simulink model "mpc_tmpdemo2"  (R2015a)
settings: Solver=ode45  SolverMode=SingleTasking  StartTime=0.0  StopTime=20.0  RelTol=1e-3
PreLoadFcn:
  | load mpc_tmpdemodata;
  | mpctmpinit
undefined symbols (not defined in the file or in its folder): Fb0, Fbh0, iA, ke, ke2, kf, kf2, lastu, lastx, m2, M2, MVscale, nv, nym, p, Rscale, st, ts, uoff, xoff
libraries: mpcsigdimcheck_private x14, cstblocks x9, simulink x4
settings Model: FPTRunName=Active  CovSFcnEnable=off  Creator=The MathWorks Inc.  LastModifiedBy=Yi
settings OptimizationCC: BlockReduction=off  BooleanDataType=off
settings DebuggingCC: SaveWithParameterizedLinksMsg=none  UnderspecifiedInitializationDetection=Classic  MergeDetectMultiDrivingBlocksExec=none  SignalResolutionControl=TryResolveAllWithWarning
settings HardwareCC: TargetUnknown=on

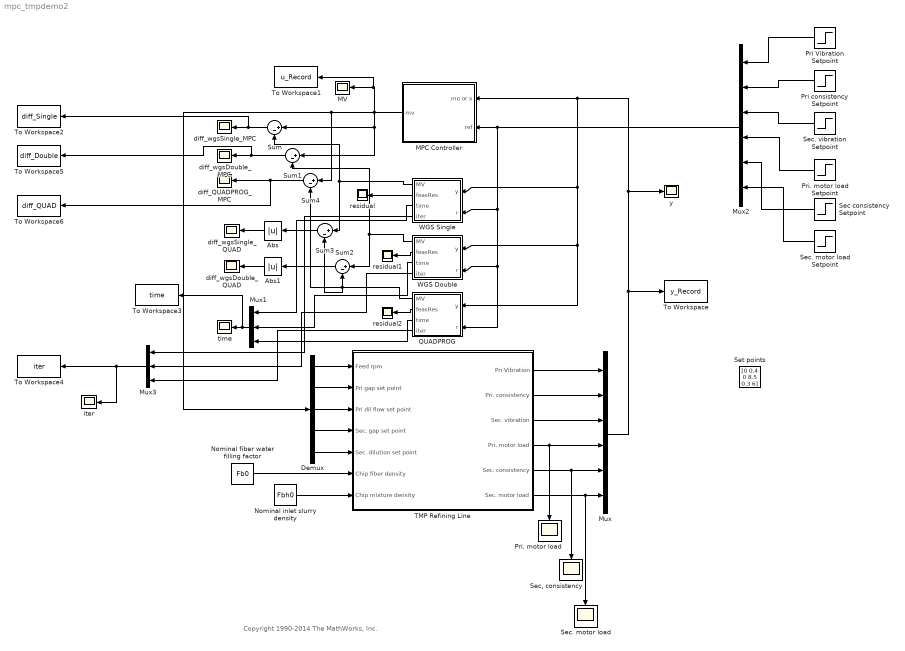
== system mpc_tmpdemo2 ==
  note: Copyright 1990-2014 The MathWorks, Inc.
  " residual" : Scope
      settings: TimeRange=7  YMin=-0.05  YMax=0.15  SaveName=ScopeData4  DataFormat=Structure
  " residual1" : Scope
      settings: TimeRange=7  YMin=-0.05  YMax=0.15  SaveName=ScopeData9  DataFormat=Structure
  " residual2" : Scope
      settings: TimeRange=7  YMin=-0.05  YMax=0.15  SaveName=ScopeData10  DataFormat=Structure
  Abs : Abs
  Abs1 : Abs
  Demux : Demux  Outputs=5
  MPC Controller : Subsystem  AncestorBlock=mpclib/MPC Controller  InitFcn=impcblock_InitFcn  StartFcn=impcblock_StartFcn  mask(MPC){mpcobj=mpcobj, x0=[], is_multiple=0, enable_value=0, n_mv=5, n_mo=6, n_md=0, n_ts=0.5, is_designfromscratch=0, return_u0=off, ref_from_ws=off, ref_signal_name=[], ref_preview=on, md_from_ws=off, md_signal_name=[], md_preview=on, from_project=off, project_file=MPCtask.mat, project_name=, task_name=, md_inport=off, mv_inport=off, cost_outport=off, return_sequence=off, return_qpstatus=off, return_state=off, state_inport=off, lims_inport=off, ywt_inport=off, uwt_inport=off, duwt_inport=off, rhoeps_inport=off, uref_inport=off, BlockDataType=double, SampleTimeInherited=off, switch_inport=off}
      mask prompts: mpcobj "MPC:general:BlgIMPC"; x0 "MPC:general:BlgState"; is_multiple "Flag indicating the block is part of multiple blocks"; enable_value "Value enabling optimization"; n_mv "Number of MVs"; n_mo "Number of MOs"; n_md "Number of MDs"; n_ts "Sample Time"; is_designfromscratch "Design from scratch flag"; return_u0 "Export u0"; ref_from_ws "Obsolete"; ref_signal_name "Obsolete"; ref_preview "Obsolete"; md_from_ws "Obsolete"; md_signal_name "Obsolete"; md_preview "Obsolete"; from_project "Obsolete"; project_file "Obsolete"; project_name "Obsolete"; task_name "Obsolete"; md_inport "MPC:general:BlgMD"; mv_inport "MPC:general:BlgEXTMV"; cost_outport "MPC:general:BlgCOST"; return_sequence "MPC:general:BlgMVSEQ"; return_qpstatus "MPC:general:BlgQPSTATUS"; return_state "MPC:general:BlgESTSTATE"; state_inport "MPC:general:BlgXKK"; lims_inport "MPC:general:BlgLIMITS"; ywt_inport "MPC:general:BlgYWT"; uwt_inport "MPC:general:BlgUWT"; duwt_inport "MPC:general:BlgDUWT"; rhoeps_inport "MPC:general:BlgECRWT"; uref_inport "MPC:general:BlgMVTARGET"; BlockDataType "MPC:general:BlgDATATYPE"; SampleTimeInherited "MPC:general:BlgTS"; switch_inport "MPC:general:BlgSWITCH"
      mask help: MPC:utility:MaskDescMPC1
      mask init:
      | [blk,ts,A,Cm,Bu,Bv,Dvm,isQP,strmoorx,nmoorx,nu,nv,ny,nx,nym...
      |     degrees,L,M,H,Hinv,Linv,iA,Ac,Kx,Ku1,Kut,Kr,Kv,...
      |     Mlim,Mx,Mu1,Mv,z_degrees,utarget,...
      |     lastx,lastu,p,xoff,uoff,yoff,voff,myoff,no_md,no_ref,...
      |     maxiter,nxQP,openloopflag,no_ym,...
      |     lims_inport,no_umin,no_umax,no_ymin,no_ymax,...
      |     switch_inport,no_switch,enable_value,...
      |     return_cost,return_sequence,CustomEstimation,...
      |     no_ywt, no_uwt, no_duwt, no_rhoeps, no_uref, no_mv, ...
      |     Wy,Wdu,Jm,SuJm,Su1,Sx,Hv,Wu,I1,...
      |     isAdaptive, C, Dv, Mrows, nCC, Ecc, Fcc, Scc, Gcc, ...
      |     Uscale, Yscale, nxp, nxindist, mvindex, mdindex, unindex,  ...
      |     myindex,Rscale,MVscale,MDscale] = impcblock_MaskInitFcnParameter();
      | impcblock_MaskInitFcnResize(gcb,nv,nu,ny);
      settings: DeleteFcn=impcblock_DeleteFcn
      mask Help: eval('mpcCSHelp(''MPCmask'',''HelpBrowser'')');
      mask Callback state_inport: mpc_blockdialogcallback(gcb);
      mask DialogControl design_button Prompt: MPC:general:BlgDesignButton
      mask DialogControl design_button Callback: mpc_designcallback(gcbh)
      mask DialogControl review_button Prompt: MPC:general:BlgReviewButton
      mask DialogControl review_button Callback: mpc_reviewcallback(gcbh)
      mask Display:
      | fprintf('MPC');
      | port_label('output', 1, 'mv')
      | port_label('input', 1, 'mo')
      | port_label('input', 2, 'ref')
  MV : Scope
      settings: SaveName=ScopeData6
  Mux : Mux  Inputs=6
  Mux1 : Mux  Inputs=3
  Mux2 : Mux  Inputs=6
  Mux3 : Mux  Inputs=3
  Nominal fiber water filling factor : Constant  Value=Fb0
  Nominal inlet slurry density : Constant  Value=Fbh0
  Pri Vibration Setpoint : Step  Time=0  After=0  SampleTime=0
  Pri consistency Setpoint : Step  Before=0.5  After=0.5  SampleTime=0
  Pri. motor load : Scope
      settings: YMin=0.3825  YMax=0.415
  Pri. motor load Setpoint : Step  Time=0  Before=8.5  After=8.5  SampleTime=0
  QUADPROG : Subsystem
  Sec consistency Setpoint : Step  Time=0  Before=0.4  After=0.4  SampleTime=0
  "Sec, consistency" : Scope
      settings: YMin=0.3825  YMax=0.415
  Sec. motor load : Scope
      settings: YMin=0.3825  YMax=0.415  SaveName=ScopeData2
  Sec. motor load Setpoint : Step  Time=0  Before=7  After=7  SampleTime=0
  Sec. vibration Setpoint : Step  Time=0  After=0  SampleTime=0
  Set points : Constant  Value=[0 0.4 0 8.5 0.3 6]
  Sum{,1..4} (5 alike) : Sum  Inputs=|+-
  TMP Refining Line : Subsystem
  To Workspace : ToWorkspace  VariableName=y_Record  SampleTime=-1
  To Workspace1 : ToWorkspace  VariableName=u_Record  SampleTime=-1
  To Workspace2 : ToWorkspace  VariableName=diff_Single  SampleTime=-1
  To Workspace3 : ToWorkspace  VariableName=time  SampleTime=-1
  To Workspace4 : ToWorkspace  VariableName=iter  SampleTime=-1
  To Workspace5 : ToWorkspace  VariableName=diff_Double  SampleTime=-1
  To Workspace6 : ToWorkspace  VariableName=diff_QUAD  SampleTime=-1
  WGS Double : Subsystem
  WGS Single : Subsystem
  diff_QUADPROG_MPC : Scope
      settings: SaveName=ScopeData14
  diff_wgsDouble_MPC : Scope
      settings: SaveName=ScopeData5
  diff_wgsDouble_QUAD : Scope
      settings: SaveName=ScopeData11
  diff_wgsSingle_MPC : Scope
      settings: SaveName=ScopeData3
  diff_wgsSingle_QUAD : Scope
      settings: SaveName=ScopeData12
  iter : Scope
      settings: SaveName=ScopeData16
  time : Scope
      settings: SaveName=ScopeData13
  y : Scope
      settings: SaveName=ScopeData15
  wires:
  Demux/1 -> TMP Refining Line/1(Feed rpm)
  Demux/3 -> TMP Refining Line/3(Pri dil flow set point)
  Demux/4 -> TMP Refining Line/4(Sec. gap set point)
  Demux/5 -> TMP Refining Line/5(Sec. dilution set point)
  TMP Refining Line/1(Pri Vibration) -> Mux/1
  TMP Refining Line/2(Pri. consistency) -> Mux/2
  TMP Refining Line/3(Sec. vibration) -> Mux/3
  TMP Refining Line/4(Pri. motor load) -> Mux/4, Pri. motor load/1
  TMP Refining Line/5(Sec. consistency) -> Mux/5, "Sec, consistency"/1
  TMP Refining Line/6(Sec. motor load) -> Mux/6, Sec. motor load/1
  Mux/1 -> To Workspace/1, y/1, MPC Controller/1(mo or x), WGS Single/1(y), WGS Double/1(y), QUADPROG/1(y)
  Mux2/1 -> WGS Double/2(r), QUADPROG/2(r), WGS Single/2(r), MPC Controller/2(ref)
  Demux/2 -> TMP Refining Line/2(Pri gap set point)
  Nominal fiber water filling factor/1 -> TMP Refining Line/6(Chip fiber density)
  MPC Controller/1(mv) -> Sum1/1, Sum/1, To Workspace1/1, MV/1, Sum4/1, Demux/1
  Nominal inlet slurry density/1 -> TMP Refining Line/7(Chip mixture density)
  Sum/1 -> To Workspace2/1, diff_wgsSingle_MPC/1
  WGS Single/2(feasRes) -> " residual"/1
  WGS Single/1(MV) -> Sum3/1, Sum/2
  WGS Double/1(MV) -> Sum2/1, Sum1/2
  Sum1/1 -> To Workspace5/1, diff_wgsDouble_MPC/1
  WGS Double/2(feasRes) -> " residual1"/1
  QUADPROG/2(feasRes) -> " residual2"/1
  QUADPROG/1(MV) -> Sum3/2, Sum4/2, Sum2/2
  Sum2/1 -> Abs1/1
  Sum3/1 -> Abs/1
  Abs/1 -> diff_wgsSingle_QUAD/1
  Abs1/1 -> diff_wgsDouble_QUAD/1
  WGS Double/3(time) -> Mux1/2
  WGS Single/3(time) -> Mux1/1
  Mux1/1 -> To Workspace3/1, time/1
  QUADPROG/3(time) -> Mux1/3
  Sum4/1 -> To Workspace6/1, diff_QUADPROG_MPC/1
  WGS Single/4(iter) -> Mux3/1
  WGS Double/4(iter) -> Mux3/2
  QUADPROG/4(iter) -> Mux3/3
  Mux3/1 -> iter/1, To Workspace4/1
  Pri Vibration Setpoint/1 -> Mux2/1
  Pri consistency Setpoint/1 -> Mux2/2
  Sec. vibration Setpoint/1 -> Mux2/3
  Pri. motor load Setpoint/1 -> Mux2/4
  Sec consistency Setpoint/1 -> Mux2/5
  Sec. motor load Setpoint/1 -> Mux2/6

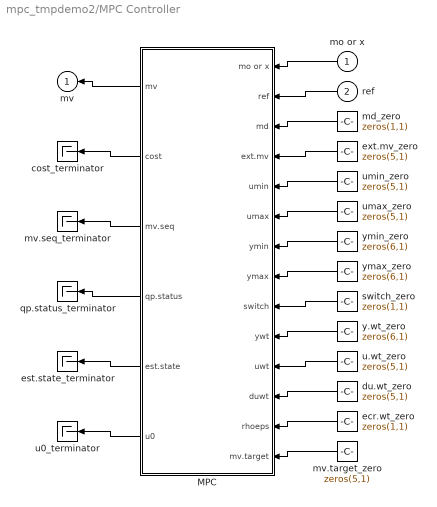
== system mpc_tmpdemo2/MPC Controller ==
  mo or x : Inport
  ref : Inport  Port=2
  MPC : Subsystem
  cost_terminator : Terminator
  du.wt_zero : Constant  Value=zeros(5,1)  OutDataTypeStr=BlockDataType
  ecr.wt_zero : Constant  Value=zeros(1,1)  OutDataTypeStr=BlockDataType
  est.state_terminator : Terminator
  ext.mv_zero : Constant  Value=zeros(5,1)  OutDataTypeStr=BlockDataType
  md_zero : Constant  Value=zeros(1,1)  OutDataTypeStr=BlockDataType
  mv.seq_terminator : Terminator
  mv.target_zero : Constant  Value=zeros(5,1)  OutDataTypeStr=BlockDataType
  qp.status_terminator : Terminator
  switch_zero : Constant  Value=zeros(1,1)  OutDataTypeStr=BlockDataType
  u.wt_zero : Constant  Value=zeros(5,1)  OutDataTypeStr=BlockDataType
  u0_terminator : Terminator
  umax_zero : Constant  Value=zeros(5,1)  OutDataTypeStr=BlockDataType
  umin_zero : Constant  Value=zeros(5,1)  OutDataTypeStr=BlockDataType
  y.wt_zero : Constant  Value=zeros(6,1)  OutDataTypeStr=BlockDataType
  ymax_zero : Constant  Value=zeros(6,1)  OutDataTypeStr=BlockDataType
  ymin_zero : Constant  Value=zeros(6,1)  OutDataTypeStr=BlockDataType
  mv : Outport
  wires:
  ext.mv_zero/1 -> MPC/4(ext.mv)
  MPC/5(est.state) -> est.state_terminator/1
  MPC/6(u0) -> u0_terminator/1
  ymax_zero/1 -> MPC/8(ymax)
  ymin_zero/1 -> MPC/7(ymin)
  umax_zero/1 -> MPC/6(umax)
  umin_zero/1 -> MPC/5(umin)
  switch_zero/1 -> MPC/9(switch)
  mv.target_zero/1 -> MPC/14(mv.target)
  u.wt_zero/1 -> MPC/11(uwt)
  MPC/4(qp.status) -> qp.status_terminator/1
  MPC/3(mv.seq) -> mv.seq_terminator/1
  MPC/2(cost) -> cost_terminator/1
  ecr.wt_zero/1 -> MPC/13(rhoeps)
  du.wt_zero/1 -> MPC/12(duwt)
  y.wt_zero/1 -> MPC/10(ywt)
  MPC/1(mv) -> mv/1
  mo or x/1 -> MPC/1(mo or x)
  ref/1 -> MPC/2(ref)
  md_zero/1 -> MPC/3(md)

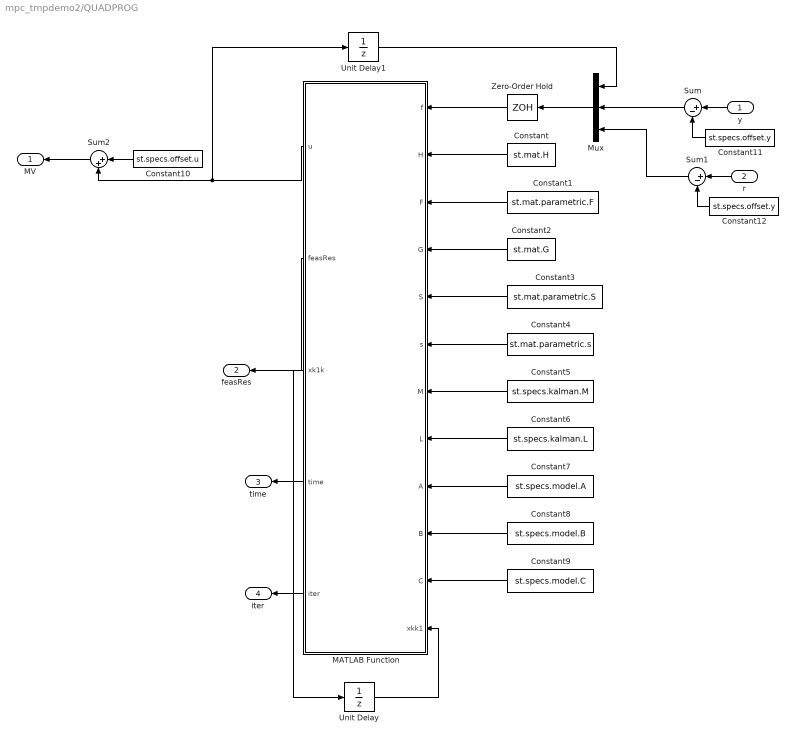
== system mpc_tmpdemo2/QUADPROG ==
  y : Inport
  r : Inport  Port=2
  Constant : Constant  Value=st.mat.H
  Constant1 : Constant  Value=st.mat.parametric.F
  Constant10 : Constant  Value=st.specs.offset.u
  Constant11 : Constant  Value=st.specs.offset.y
  Constant12 : Constant  Value=st.specs.offset.y
  Constant2 : Constant  Value=st.mat.G
  Constant3 : Constant  Value=st.mat.parametric.S
  Constant4 : Constant  Value=st.mat.parametric.s
  Constant5 : Constant  Value=st.specs.kalman.M
  Constant6 : Constant  Value=st.specs.kalman.L
  Constant7 : Constant  Value=st.specs.model.A
  Constant8 : Constant  Value=st.specs.model.B
  Constant9 : Constant  Value=st.specs.model.C
  MATLAB Function : MATLAB Function  TreatAsAtomicUnit=on
  Mux : Mux  Inputs=3
  Sum : Sum  Inputs=|+-
  Sum1 : Sum  Inputs=|+-
  Sum2 : Sum  Inputs=|++
  Unit Delay : UnitDelay  InitialCondition=st.specs.init.x0  SampleTime=st.specs.model.Ts
  Unit Delay1 : UnitDelay  InitialCondition=st.specs.init.u0  SampleTime=st.specs.model.Ts
  Zero-Order Hold : ZeroOrderHold  SampleTime=st.specs.model.Ts
  MV : Outport
  feasRes : Outport  Port=2
  time : Outport  Port=3
  iter : Outport  Port=4
  wires:
  Sum2/1 -> MV/1
  Constant10/1 -> Sum2/1
  r/1 -> Sum1/1
  Sum1/1 -> Mux/3
  Constant12/1 -> Sum1/2
  y/1 -> Sum/1
  Sum/1 -> Mux/2
  Constant11/1 -> Sum/2
  Unit Delay1/1 -> Mux/1
  Mux/1 -> Zero-Order Hold/1
  MATLAB Function/2(feasRes) -> feasRes/1
  Constant9/1 -> MATLAB Function/11(C)
  MATLAB Function/3(xk1k) -> Unit Delay/1
  Zero-Order Hold/1 -> MATLAB Function/1(f)
  Constant/1 -> MATLAB Function/2(H)
  Constant1/1 -> MATLAB Function/3(F)
  Constant2/1 -> MATLAB Function/4(G)
  Constant3/1 -> MATLAB Function/5(S)
  Constant4/1 -> MATLAB Function/6(s)
  Constant5/1 -> MATLAB Function/7(M)
  Constant6/1 -> MATLAB Function/8(L)
  Constant7/1 -> MATLAB Function/9(A)
  Constant8/1 -> MATLAB Function/10(B)
  MATLAB Function/1(u) -> Sum2/2, Unit Delay1/1
  Unit Delay/1 -> MATLAB Function/12(xkk1)
  MATLAB Function/4(time) -> time/1
  MATLAB Function/5(iter) -> iter/1

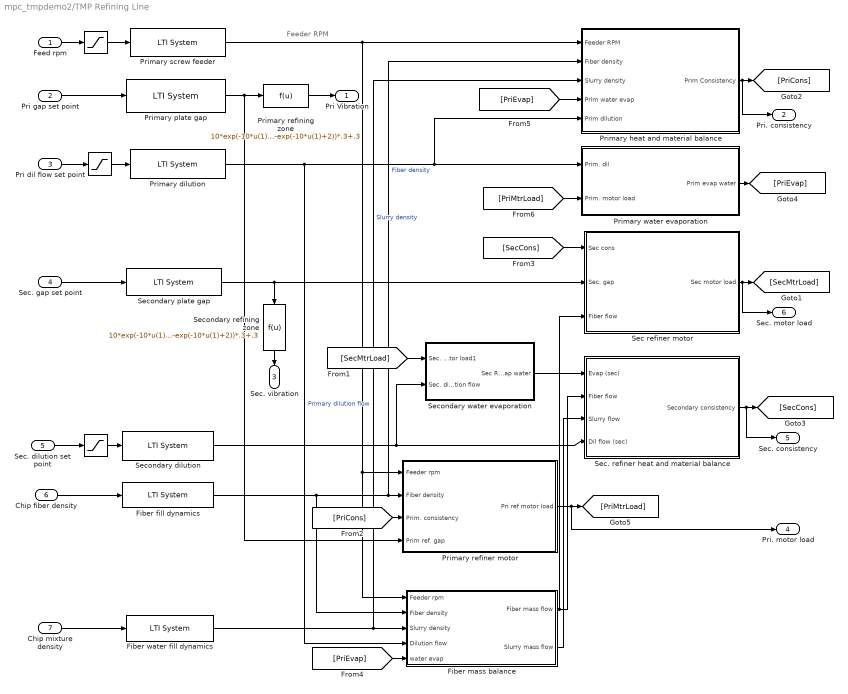
== system mpc_tmpdemo2/TMP Refining Line ==
  note: Feeder RPM
  Feed rpm : Inport
  Pri gap set point : Inport  Port=2
  Pri dil flow set point : Inport  Port=3
  Sec. gap set point : Inport  Port=4
  Sec. dilution set point : Inport  Port=5
  Chip fiber density : Inport  Port=6
  Chip mixture density : Inport  Port=7
  "  " : Saturate  UpperLimit=35  LowerLimit=25  SampleTime=0.5
  "    " : Saturate  UpperLimit=200  LowerLimit=90  SampleTime=0.5
  "       " : Saturate  UpperLimit=200  LowerLimit=90  SampleTime=0.5
  Fiber fill dynamics : cstblocks/LTI System  sys=FiberFill  IC=Fb0
  Fiber mass balance : Subsystem
  Fiber water fill dynamics : cstblocks/LTI System  sys=FiberWaterFill  IC=Fbh0
  Primary dilution : cstblocks/LTI System  sys=DilFlowPrimary  IC=dp0
  Primary heat and material balance : Subsystem
  Primary plate gap : cstblocks/LTI System  sys=PlateGapPrimary  IC=gp0
  Primary refiner motor : Subsystem
  Primary refining zone : Fcn  Expr=10*exp(-10*u(1)+2)*(1.26-0.3*u(1))-(1-exp(-10*u(1)+2))*.3+.3
  Primary screw feeder : cstblocks/LTI System  sys=ChipFeeder  IC=vp0
  Primary water evaporation : Subsystem
  Sec refiner motor : Subsystem
  Sec. refiner heat and material balance : Subsystem
  "Secondary dilution " : cstblocks/LTI System  sys=DilFlowSecondary  IC=gs0
  Secondary plate gap : cstblocks/LTI System  sys=PlateGapSecondary  IC=gs0
  Secondary refining zone : Fcn  Expr=10*exp(-10*u(1)+2)*(1.26-0.3*u(1))-(1-exp(-10*u(1)+2))*.3+.3  SampleTime=0.5
  Secondary water evaporation : Subsystem
  Pri Vibration : Outport
  Pri. consistency : Outport  Port=2
  Sec. vibration : Outport  Port=3
  Pri. motor load : Outport  Port=4
  Sec. consistency : Outport  Port=5
  Sec. motor load : Outport  Port=6
  wires:
  "  "/1 -> Primary screw feeder/1
  Primary plate gap/1 -> Primary refining zone/1, Primary refiner motor/4(Prim ref. gap)
  Secondary plate gap/1 -> Secondary refining zone/1, Sec refiner motor/2(Sec. gap)
  "    "/1 -> Primary dilution/1
  "       "/1 -> "Secondary dilution "/1
  "Secondary dilution "/1 -> Sec. refiner heat and material balance/4(Dil flow (sec)), Secondary water evaporation/2(Sec. dilution flow)
  Sec. dilution set point/1 -> "       "/1
  Fiber water fill dynamics/1 -> Primary heat and material balance/3(Slurry density), Fiber mass balance/3(Slurry density)  "Slurry density"
  Fiber fill dynamics/1 -> Fiber mass balance/2(Fiber density), Primary heat and material balance/2(Fiber density), Primary refiner motor/2(Fiber density)  "Fiber density"
  Primary dilution/1 -> Primary water evaporation/1(Prim. dil), Primary heat and material balance/5(Prim dilution), Fiber mass balance/4(Dilution flow)  "Primary dilution flow"
  Primary screw feeder/1 -> Primary heat and material balance/1(Feeder RPM), Fiber mass balance/1(Feeder rpm), Primary refiner motor/1(Feeder rpm)
  Fiber mass balance/1(Fiber mass flow) -> Sec. refiner heat and material balance/2(Fiber flow), Sec refiner motor/3(Fiber flow)
  Fiber mass balance/2(Slurry mass flow) -> Sec. refiner heat and material balance/3(Slurry flow)
  Secondary water evaporation/1(Sec Ref. evap water) -> Sec. refiner heat and material balance/1(Evap (sec))
  Primary refining zone/1 -> Pri Vibration/1
  Sec refiner motor/1(Sec motor load) -> [SecMtrLoad], Sec. motor load/1
  Primary heat and material balance/1(Prim Consistency) -> [PriCons], Pri. consistency/1
  [PriCons] -> Primary refiner motor/3(Prim. consistency)
  Sec. refiner heat and material balance/1(Secondary consistency) -> [SecCons], Sec. consistency/1
  [SecCons] -> Sec refiner motor/1(Sec cons)
  Primary water evaporation/1(Prim evap water) -> [PriEvap]
  [PriEvap] -> Primary heat and material balance/4(Prim water evap)
  Primary refiner motor/1(Pri ref motor load) -> [PriMtrLoad], Pri. motor load/1
  [PriMtrLoad] -> Primary water evaporation/2(Prim. motor load)
  [SecMtrLoad] -> Secondary water evaporation/1(Sec. motor load1)
  Feed rpm/1 -> "  "/1
  Pri gap set point/1 -> Primary plate gap/1
  Pri dil flow set point/1 -> "    "/1
  Sec. gap set point/1 -> Secondary plate gap/1
  Secondary refining zone/1 -> Sec. vibration/1
  [PriEvap] -> Fiber mass balance/5(water evap)
  Chip fiber density/1 -> Fiber fill dynamics/1
  Chip mixture density/1 -> Fiber water fill dynamics/1

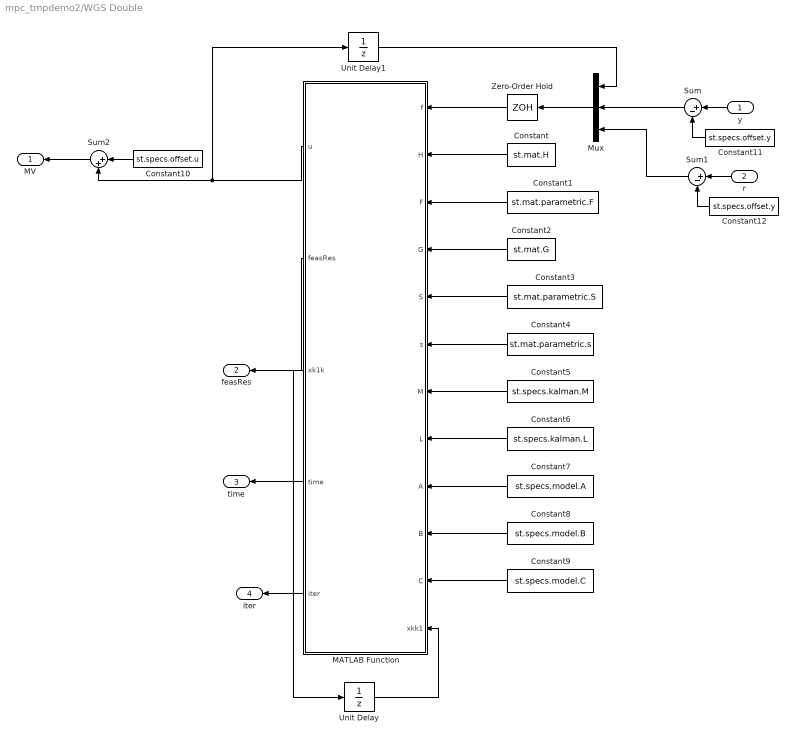
== system mpc_tmpdemo2/WGS Double ==
  y : Inport
  r : Inport  Port=2
  Constant : Constant  Value=st.mat.H
  Constant1 : Constant  Value=st.mat.parametric.F
  Constant10 : Constant  Value=st.specs.offset.u
  Constant11 : Constant  Value=st.specs.offset.y
  Constant12 : Constant  Value=st.specs.offset.y
  Constant2 : Constant  Value=st.mat.G
  Constant3 : Constant  Value=st.mat.parametric.S
  Constant4 : Constant  Value=st.mat.parametric.s
  Constant5 : Constant  Value=st.specs.kalman.M
  Constant6 : Constant  Value=st.specs.kalman.L
  Constant7 : Constant  Value=st.specs.model.A
  Constant8 : Constant  Value=st.specs.model.B
  Constant9 : Constant  Value=st.specs.model.C
  MATLAB Function : MATLAB Function  TreatAsAtomicUnit=on
  Mux : Mux  Inputs=3
  Sum : Sum  Inputs=|+-
  Sum1 : Sum  Inputs=|+-
  Sum2 : Sum  Inputs=|++
  Unit Delay : UnitDelay  InitialCondition=st.specs.init.x0  SampleTime=st.specs.model.Ts
  Unit Delay1 : UnitDelay  InitialCondition=st.specs.init.u0  SampleTime=st.specs.model.Ts
  Zero-Order Hold : ZeroOrderHold  SampleTime=st.specs.model.Ts
  MV : Outport
  feasRes : Outport  Port=2
  time : Outport  Port=3
  iter : Outport  Port=4
  wires:
  Sum2/1 -> MV/1
  Constant10/1 -> Sum2/1
  r/1 -> Sum1/1
  Sum1/1 -> Mux/3
  Constant12/1 -> Sum1/2
  y/1 -> Sum/1
  Sum/1 -> Mux/2
  Constant11/1 -> Sum/2
  Unit Delay1/1 -> Mux/1
  Mux/1 -> Zero-Order Hold/1
  MATLAB Function/2(feasRes) -> feasRes/1
  Constant9/1 -> MATLAB Function/11(C)
  MATLAB Function/3(xk1k) -> Unit Delay/1
  Zero-Order Hold/1 -> MATLAB Function/1(f)
  Constant/1 -> MATLAB Function/2(H)
  Constant1/1 -> MATLAB Function/3(F)
  Constant2/1 -> MATLAB Function/4(G)
  Constant3/1 -> MATLAB Function/5(S)
  Constant4/1 -> MATLAB Function/6(s)
  Constant5/1 -> MATLAB Function/7(M)
  Constant6/1 -> MATLAB Function/8(L)
  Constant7/1 -> MATLAB Function/9(A)
  Constant8/1 -> MATLAB Function/10(B)
  MATLAB Function/1(u) -> Sum2/2, Unit Delay1/1
  Unit Delay/1 -> MATLAB Function/12(xkk1)
  MATLAB Function/4(time) -> time/1
  MATLAB Function/5(iter) -> iter/1

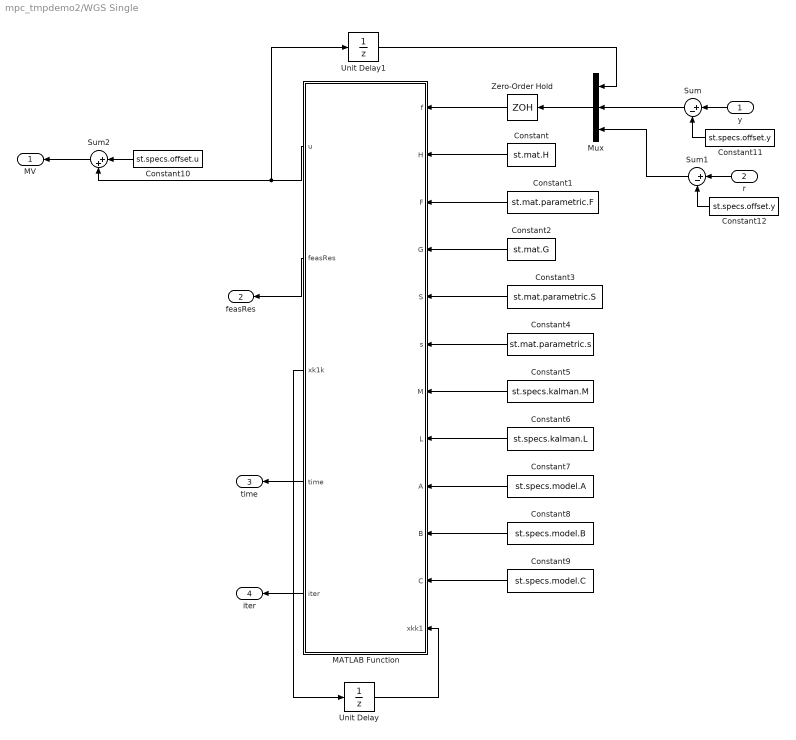
== system mpc_tmpdemo2/WGS Single ==
  y : Inport
  r : Inport  Port=2
  Constant : Constant  Value=st.mat.H
  Constant1 : Constant  Value=st.mat.parametric.F
  Constant10 : Constant  Value=st.specs.offset.u
  Constant11 : Constant  Value=st.specs.offset.y
  Constant12 : Constant  Value=st.specs.offset.y
  Constant2 : Constant  Value=st.mat.G
  Constant3 : Constant  Value=st.mat.parametric.S
  Constant4 : Constant  Value=st.mat.parametric.s
  Constant5 : Constant  Value=st.specs.kalman.M
  Constant6 : Constant  Value=st.specs.kalman.L
  Constant7 : Constant  Value=st.specs.model.A
  Constant8 : Constant  Value=st.specs.model.B
  Constant9 : Constant  Value=st.specs.model.C
  MATLAB Function : MATLAB Function  TreatAsAtomicUnit=on
  Mux : Mux  Inputs=3
  Sum : Sum  Inputs=|+-
  Sum1 : Sum  Inputs=|+-
  Sum2 : Sum  Inputs=|++
  Unit Delay : UnitDelay  InitialCondition=st.specs.init.x0  SampleTime=st.specs.model.Ts
  Unit Delay1 : UnitDelay  InitialCondition=st.specs.init.u0  SampleTime=st.specs.model.Ts
  Zero-Order Hold : ZeroOrderHold  SampleTime=st.specs.model.Ts
  MV : Outport
  feasRes : Outport  Port=2
  time : Outport  Port=3
  iter : Outport  Port=4
  wires:
  Zero-Order Hold/1 -> MATLAB Function/1(f)
  Unit Delay/1 -> MATLAB Function/12(xkk1)
  MATLAB Function/3(xk1k) -> Unit Delay/1
  Constant9/1 -> MATLAB Function/11(C)
  Constant8/1 -> MATLAB Function/10(B)
  Constant7/1 -> MATLAB Function/9(A)
  Constant6/1 -> MATLAB Function/8(L)
  Constant5/1 -> MATLAB Function/7(M)
  MATLAB Function/2(feasRes) -> feasRes/1
  Constant4/1 -> MATLAB Function/6(s)
  Constant3/1 -> MATLAB Function/5(S)
  Constant2/1 -> MATLAB Function/4(G)
  Constant1/1 -> MATLAB Function/3(F)
  Constant/1 -> MATLAB Function/2(H)
  Mux/1 -> Zero-Order Hold/1
  Unit Delay1/1 -> Mux/1
  MATLAB Function/1(u) -> Sum2/2, Unit Delay1/1
  Constant11/1 -> Sum/2
  Sum/1 -> Mux/2
  y/1 -> Sum/1
  Constant12/1 -> Sum1/2
  Sum1/1 -> Mux/3
  r/1 -> Sum1/1
  Constant10/1 -> Sum2/1
  Sum2/1 -> MV/1
  MATLAB Function/4(time) -> time/1
  MATLAB Function/5(iter) -> iter/1

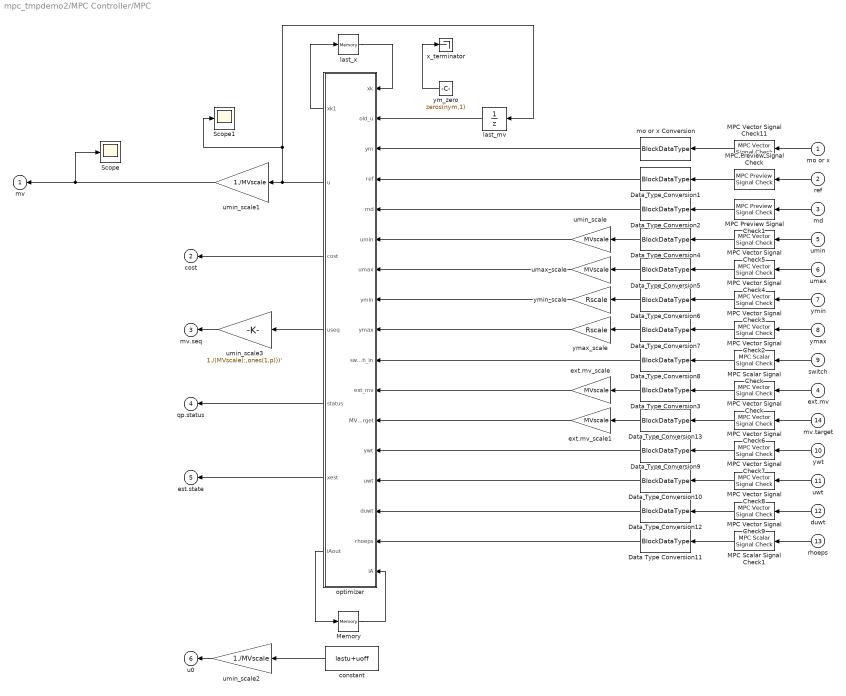
== system mpc_tmpdemo2/MPC Controller/MPC ==
  mo or x : Inport
  ref : Inport  Port=2
  md : Inport  Port=3
  ext.mv : Inport  Port=4
  umin : Inport  Port=5
  umax : Inport  Port=6
  ymin : Inport  Port=7
  ymax : Inport  Port=8
  switch : Inport  Port=9
  ywt : Inport  Port=10
  uwt : Inport  Port=11
  duwt : Inport  Port=12
  rhoeps : Inport  Port=13
  mv.target : Inport  Port=14
  Data Type Conversion{1..13} (13 alike) : DataTypeConversion  OutDataTypeStr=BlockDataType
  MPC Preview Signal Check : mpcsigdimcheck_private/MPC Preview Signal Check  blockname=blk  signalname='ref'  numrow=p  numcol=ny
  MPC Preview Signal Check1 : mpcsigdimcheck_private/MPC Preview Signal Check  blockname=blk  signalname='md'  numrow=p+1  numcol=max(nv-1,1)
  MPC Scalar Signal Check : mpcsigdimcheck_private/MPC Scalar Signal Check  blockname=blk  signalname='switch'
  MPC Scalar Signal Check1 : mpcsigdimcheck_private/MPC Scalar Signal Check  blockname=blk  signalname='ecr.wt'
  MPC Vector Signal Check : mpcsigdimcheck_private/MPC Vector Signal Check  blockname=blk  signalname='ext.mv'  num=nu  vectortype=Any
  MPC Vector Signal Check11 : mpcsigdimcheck_private/MPC Vector Signal Check  blockname=blk  signalname=strmoorx  num=nmoorx  vectortype=Any
  MPC Vector Signal Check2 : mpcsigdimcheck_private/MPC Vector Signal Check  blockname=blk  signalname='ymax'  num=ny  vectortype=Any
  MPC Vector Signal Check3 : mpcsigdimcheck_private/MPC Vector Signal Check  blockname=blk  signalname='ymin'  num=ny  vectortype=Any
  MPC Vector Signal Check4 : mpcsigdimcheck_private/MPC Vector Signal Check  blockname=blk  signalname='umax'  num=nu  vectortype=Any
  MPC Vector Signal Check5 : mpcsigdimcheck_private/MPC Vector Signal Check  blockname=blk  signalname='umin'  num=nu  vectortype=Any
  MPC Vector Signal Check6 : mpcsigdimcheck_private/MPC Vector Signal Check  blockname=blk  signalname='mv.target'  num=nu  vectortype=Any
  MPC Vector Signal Check7 : mpcsigdimcheck_private/MPC Vector Signal Check  blockname=blk  signalname='y.wt'  num=ny  vectortype=Any
  MPC Vector Signal Check8 : mpcsigdimcheck_private/MPC Vector Signal Check  blockname=blk  signalname='u.wt'  num=nu  vectortype=Any
  MPC Vector Signal Check9 : mpcsigdimcheck_private/MPC Vector Signal Check  blockname=blk  signalname='du.wt'  num=nu  vectortype=Any
  Memory : Memory  X0=iA  InheritSampleTime=on  LinearizeAsDelay=on
  Scope : Scope
      settings: SaveName=ScopeData7
  Scope1 : Scope
      settings: SaveName=ScopeData8
  constant : Constant  Value=lastu+uoff
  ext.mv_scale : Gain  Gain=MVscale  SampleTime=ts
  ext.mv_scale1 : Gain  Gain=MVscale  SampleTime=ts
  last_mv : UnitDelay  InitialCondition=lastu+uoff  SampleTime=ts
  last_x : Memory  X0=lastx+xoff  InheritSampleTime=on  LinearizeAsDelay=on
  mo or x Conversion : DataTypeConversion  OutDataTypeStr=BlockDataType
  optimizer : MATLAB Function
  umax_scale : Gain  Gain=MVscale  SampleTime=ts
  umin_scale : Gain  Gain=MVscale  SampleTime=ts
  umin_scale1 : Gain  Gain=1./MVscale  SampleTime=ts
  umin_scale2 : Gain  Gain=1./MVscale  SampleTime=ts
  umin_scale3 : Gain  Gain=1./(MVscale(:,ones(1,p)))'  SampleTime=ts
  x_terminator : Terminator
  ym_zero : Constant  Value=zeros(nym,1)  OutDataTypeStr=BlockDataType
  ymax_scale : Gain  Gain=Rscale  SampleTime=ts
  ymin_scale : Gain  Gain=Rscale  SampleTime=ts
  mv : Outport  OutDataTypeStr=BlockDataType
  cost : Outport  Port=2  OutDataTypeStr=BlockDataType
  mv.seq : Outport  Port=3  OutDataTypeStr=BlockDataType
  qp.status : Outport  Port=4  OutDataTypeStr=BlockDataType
  est.state : Outport  Port=5  OutDataTypeStr=BlockDataType
  u0 : Outport  Port=6  OutDataTypeStr=BlockDataType
  wires:
  MPC Preview Signal Check1/1 -> Data Type Conversion2/1
  MPC Preview Signal Check/1 -> Data Type Conversion1/1
  MPC Vector Signal Check11/1 -> mo or x Conversion/1
  MPC Scalar Signal Check1/1 -> Data Type Conversion11/1
  MPC Vector Signal Check9/1 -> Data Type Conversion12/1
  MPC Vector Signal Check8/1 -> Data Type Conversion10/1
  MPC Vector Signal Check7/1 -> Data Type Conversion9/1
  MPC Vector Signal Check6/1 -> Data Type Conversion13/1
  MPC Vector Signal Check5/1 -> Data Type Conversion4/1
  MPC Vector Signal Check4/1 -> Data Type Conversion5/1
  MPC Vector Signal Check3/1 -> Data Type Conversion6/1
  MPC Vector Signal Check2/1 -> Data Type Conversion7/1
  MPC Scalar Signal Check/1 -> Data Type Conversion8/1
  MPC Vector Signal Check/1 -> Data Type Conversion3/1
  ym_zero/1 -> x_terminator/1
  last_x/1 -> optimizer/1(xk)
  mo or x Conversion/1 -> optimizer/3(ym)
  optimizer/6(xest) -> est.state/1
  umin_scale3/1 -> mv.seq/1
  umin_scale1/1 -> Scope/1, mv/1
  umin_scale2/1 -> u0/1
  constant/1 -> umin_scale2/1
  ext.mv_scale/1 -> optimizer/11(ext_mv)
  optimizer/2(u) -> umin_scale1/1, last_mv/1, Scope1/1
  Data Type Conversion1/1 -> optimizer/4(ref)
  ext.mv_scale1/1 -> optimizer/12(MVtarget)
  Data Type Conversion13/1 -> ext.mv_scale1/1
  mv.target/1 -> MPC Vector Signal Check6/1
  optimizer/1(xk1) -> last_x/1
  Data Type Conversion10/1 -> optimizer/14(uwt)
  duwt/1 -> MPC Vector Signal Check9/1
  rhoeps/1 -> MPC Scalar Signal Check1/1
  Data Type Conversion2/1 -> optimizer/5(md)
  ymax_scale/1 -> optimizer/9(ymax)
  ymin_scale/1 -> optimizer/8(ymin)
  Data Type Conversion6/1 -> ymin_scale/1
  umax_scale/1 -> optimizer/7(umax)
  umin_scale/1 -> optimizer/6(umin)
  Data Type Conversion11/1 -> optimizer/16(rhoeps)
  Data Type Conversion12/1 -> optimizer/15(duwt)
  Data Type Conversion9/1 -> optimizer/13(ywt)
  Data Type Conversion8/1 -> optimizer/10(switch_in)
  Data Type Conversion7/1 -> ymax_scale/1
  Data Type Conversion5/1 -> umax_scale/1
  Data Type Conversion4/1 -> umin_scale/1
  uwt/1 -> MPC Vector Signal Check8/1
  ywt/1 -> MPC Vector Signal Check7/1
  optimizer/7(iAout) -> Memory/1
  optimizer/5(status) -> qp.status/1
  Memory/1 -> optimizer/17(iA)
  ref/1 -> MPC Preview Signal Check/1
  last_mv/1 -> optimizer/2(old_u)
  Data Type Conversion3/1 -> ext.mv_scale/1
  ext.mv/1 -> MPC Vector Signal Check/1
  switch/1 -> MPC Scalar Signal Check/1
  ymax/1 -> MPC Vector Signal Check2/1
  ymin/1 -> MPC Vector Signal Check3/1
  umax/1 -> MPC Vector Signal Check4/1
  umin/1 -> MPC Vector Signal Check5/1
  md/1 -> MPC Preview Signal Check1/1
  optimizer/3(cost) -> cost/1
  optimizer/4(useq) -> umin_scale3/1
  mo or x/1 -> MPC Vector Signal Check11/1

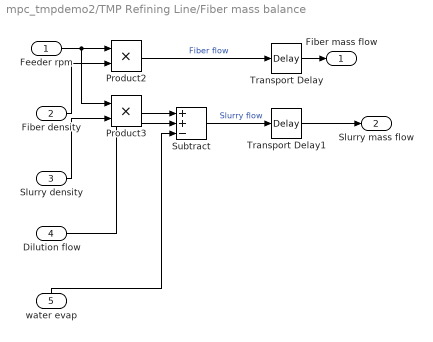
== system mpc_tmpdemo2/TMP Refining Line/Fiber mass balance ==
  Feeder rpm : Inport
  Fiber density : Inport  Port=2
  Slurry density : Inport  Port=3
  Dilution flow : Inport  Port=4
  water evap : Inport  Port=5
  Product2 : Product  RndMeth=Zero
  Product3 : Product  RndMeth=Zero
  Subtract : Sum  Inputs=++-
  Transport Delay : TransportDelay  DelayTime=2  InitialOutput=m2
  Transport Delay1 : TransportDelay  DelayTime=2  InitialOutput=M2
  Fiber mass flow : Outport
  Slurry mass flow : Outport  Port=2
  wires:
  Product2/1 -> Transport Delay/1  "Fiber flow"
  Product3/1 -> Subtract/1
  Subtract/1 -> Transport Delay1/1  "Slurry flow"
  Feeder rpm/1 -> Product2/1, Product3/1
  Fiber density/1 -> Product2/2
  Slurry density/1 -> Product3/2
  Dilution flow/1 -> Subtract/2
  water evap/1 -> Subtract/3
  Transport Delay/1 -> Fiber mass flow/1
  Transport Delay1/1 -> Slurry mass flow/1

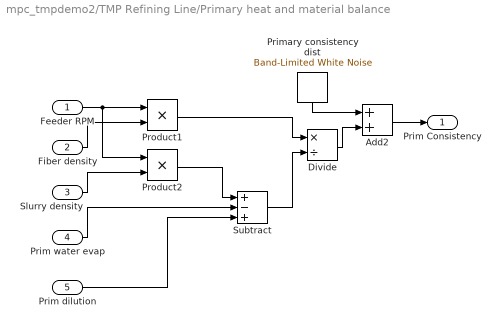
== system mpc_tmpdemo2/TMP Refining Line/Primary heat and material balance ==
  Feeder RPM : Inport
  Fiber density : Inport  Port=2
  Slurry density : Inport  Port=3
  Prim water evap : Inport  Port=4
  Prim dilution : Inport  Port=5
  Add2 : Sum
  Divide : Product  Inputs=*/  SampleTime=.5
  Primary consistency dist : simulink/Sources/Band-Limited White Noise  Cov=0.00001  Ts=0.5  seed=[23341]
  Product1 : Product  RndMeth=Zero
  Product2 : Product  RndMeth=Zero
  Subtract : Sum  Inputs=+-+
  Prim Consistency : Outport
  wires:
  Product2/1 -> Subtract/1
  Subtract/1 -> Divide/2
  Product1/1 -> Divide/1
  Divide/1 -> Add2/2
  Primary consistency dist/1 -> Add2/1
  Feeder RPM/1 -> Product1/1, Product2/1
  Prim dilution/1 -> Subtract/3
  Add2/1 -> Prim Consistency/1
  Fiber density/1 -> Product1/2
  Slurry density/1 -> Product2/2
  Prim water evap/1 -> Subtract/2

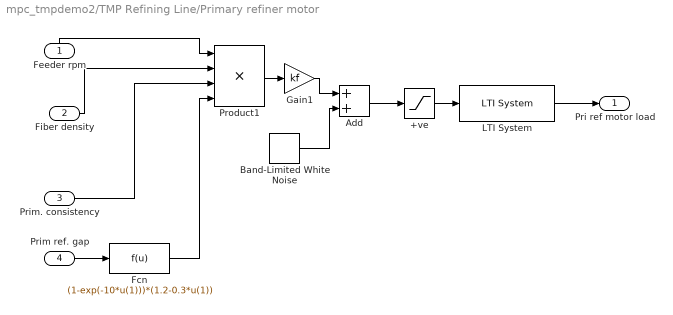
== system mpc_tmpdemo2/TMP Refining Line/Primary refiner motor ==
  Feeder rpm : Inport
  Fiber density : Inport  Port=2
  Prim. consistency : Inport  Port=3
  Prim ref. gap : Inport  Port=4
  +ve : Saturate  UpperLimit=inf  LowerLimit=0  SampleTime=0.5
  Add : Sum
  Band-Limited White Noise : simulink/Sources/Band-Limited White Noise  Cov=0.0001  Ts=0.5  seed=[23341]
  Fcn : Fcn  Expr=(1-exp(-10*u(1)))*(1.2-0.3*u(1))
  Gain1 : Gain  Gain=kf
  LTI System : cstblocks/LTI System  sys=UnitDelay  IC=mlp0
  Product1 : Product  Inputs=4  RndMeth=Zero
  Pri ref motor load : Outport
  wires:
  Product1/1 -> Gain1/1
  Fcn/1 -> Product1/4
  Gain1/1 -> Add/1
  Add/1 -> +ve/1
  Band-Limited White Noise/1 -> Add/2
  Feeder rpm/1 -> Product1/1
  Fiber density/1 -> Product1/2
  Prim ref. gap/1 -> Fcn/1
  Prim. consistency/1 -> Product1/3
  +ve/1 -> LTI System/1
  LTI System/1 -> Pri ref motor load/1

== system mpc_tmpdemo2/TMP Refining Line/Primary water evaporation ==
  Prim. dil : Inport
  Prim. motor load : Inport  Port=2
  Evap coeff (prim) : Constant  Value=ke
  Gain : Gain  Gain=1.1
  MinMax : MinMax  Inputs=2
  prim evap water : Product  RndMeth=Zero
  Prim evap water : Outport
  wires:
  Evap coeff (prim)/1 -> prim evap water/1
  prim evap water/1 -> MinMax/2
  Gain/1 -> MinMax/1
  Prim. dil/1 -> Gain/1
  MinMax/1 -> Prim evap water/1  "Primary evaporated water"
  Prim. motor load/1 -> prim evap water/2

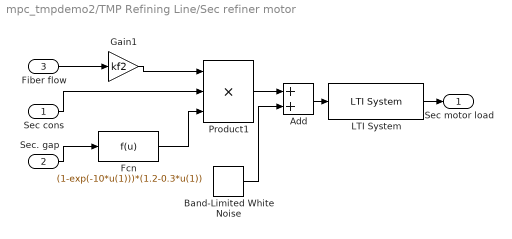
== system mpc_tmpdemo2/TMP Refining Line/Sec refiner motor ==
  Sec cons : Inport
  Sec. gap : Inport  Port=2
  Fiber flow : Inport  Port=3
  Add : Sum
  Band-Limited White Noise : simulink/Sources/Band-Limited White Noise  Cov=0.0001  Ts=0.5  seed=[23341]
  Fcn : Fcn  Expr=(1-exp(-10*u(1)))*(1.2-0.3*u(1))
  Gain1 : Gain  Gain=kf2
  LTI System : cstblocks/LTI System  sys=UnitDelay  IC=mls0
  Product1 : Product  Inputs=3  RndMeth=Zero
  Sec motor load : Outport
  wires:
  Gain1/1 -> Product1/1
  Fcn/1 -> Product1/3
  Product1/1 -> Add/1
  Band-Limited White Noise/1 -> Add/2
  Fiber flow/1 -> Gain1/1
  Sec. gap/1 -> Fcn/1
  Sec cons/1 -> Product1/2
  Add/1 -> LTI System/1
  LTI System/1 -> Sec motor load/1

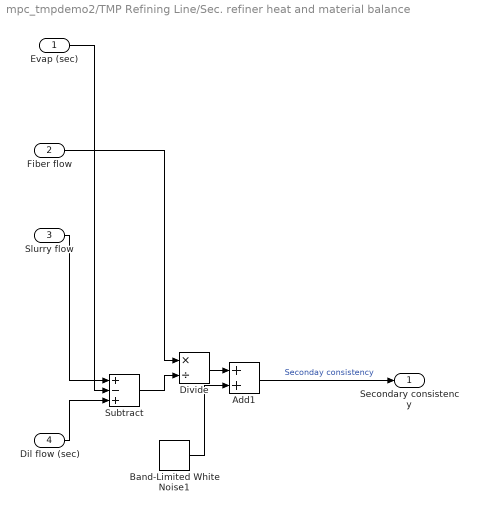
== system mpc_tmpdemo2/TMP Refining Line/Sec. refiner heat and material balance ==
  Evap (sec) : Inport
  Fiber flow : Inport  Port=2
  Slurry flow : Inport  Port=3
  Dil flow (sec) : Inport  Port=4
  Add1 : Sum
  Band-Limited White Noise1 : simulink/Sources/Band-Limited White Noise  Cov=0.00001  Ts=0.5  seed=[23341]
  Divide : Product  Inputs=*/  SampleTime=.5
  Subtract : Sum  Inputs=+-+
  Secondary consistency : Outport
  wires:
  Evap (sec)/1 -> Subtract/2
  Subtract/1 -> Divide/2
  Divide/1 -> Add1/1
  Band-Limited White Noise1/1 -> Add1/2
  Fiber flow/1 -> Divide/1
  Dil flow (sec)/1 -> Subtract/3
  Add1/1 -> Secondary consistency/1  "Seconday consistency"
  Slurry flow/1 -> Subtract/1

== system mpc_tmpdemo2/TMP Refining Line/Secondary water evaporation ==
  Sec. motor load1 : Inport
  Sec. dilution flow : Inport  Port=2
  Evap coeff (sec) : Constant  Value=ke2
  Gain1 : Gain  Gain=1.1
  MinMax1 : MinMax  Inputs=2
  prim evap water1 : Product  RndMeth=Zero
  Sec Ref. evap water : Outport
  wires:
  Evap coeff (sec)/1 -> prim evap water1/1
  prim evap water1/1 -> MinMax1/2
  Sec. dilution flow/1 -> Gain1/1
  Sec. motor load1/1 -> prim evap water1/2
  Gain1/1 -> MinMax1/1
  MinMax1/1 -> Sec Ref. evap water/1  "Secondary evaporated water"

== matlab function mpc_tmpdemo2/WGS Single/MATLAB Function ==
  data: f input; H input; F input; G input; S input; s input; u output; feasRes output; M input; L input; xk1k output; A input; B input; C input; xkk1 input; time output; iter output
%% solve the problem
%   min 0.5 z'Hz + h'z
%   s.t. Gz <= b

function [u,feasRes,xk1k,time,iter]=fcn(f,H,F,G,S,s,M,L,A,B,C,xkk1)
%% init
coder.extrinsic('quadprog');
coder.extrinsic('wgsSolver');
options.Algorithm='interior-point-convex';
options.MaxIter=1000;
options.TolCon=1.0000e-12; % default: 1e-8
options.TolFun=1.0000e-12; % default: 1e-8
options.TolX=1.0000e-12;   % default: 1e-8
options.Display='none';
zopt=zeros(size(H,1),1);
time = 0;
iter = 0;

%% get info
[~,nu]=size(B);
ny=size(C,1);
u0=f(1:nu);
y=f(nu+1:nu+ny);

xkk=xkk1+M*(y-C*xkk1);  % kalman

%% solver
p=[f(1:nu);xkk;f(ny+nu+1:2*ny+nu)];

b=S*p+s;
h=F*p;
%[zopt]=quadprog(H,h,G,b,[],[],[],[],[],options); % solve the optimal control problem
[zopt,time,iter] = wgsSolver(H,h,-G,-b,[],[],[],[],[],1);   
feasRes=G*zopt-b;

nu=length(u0);
u=zopt(1:nu)+u0;

time = double(time);

xk1k=A*xkk1+B*u+L*(y-C*xkk1); % kalman

== matlab function mpc_tmpdemo2/WGS Double/MATLAB Function ==
  data: f input; H input; F input; G input; S input; s input; u output; feasRes output; M input; L input; xk1k output; A input; B input; C input; xkk1 input; time output; iter output
%% solve the problem
%   min 0.5 z'Hz + h'z
%   s.t. Gz <= b

function [u,feasRes,xk1k,time,iter]=fcn(f,H,F,G,S,s,M,L,A,B,C,xkk1)

%% init
coder.extrinsic('quadprog');
coder.extrinsic('wgsSolver');
options.Algorithm='interior-point-convex';
options.MaxIter=1000;
options.TolCon=1.0000e-12; % default: 1e-8
options.TolFun=1.0000e-12; % default: 1e-8
options.TolX=1.0000e-12;   % default: 1e-8
options.Display='none';
zopt=zeros(size(H,1),1);
time = 0;
iter = 0;

%% get info
[~,nu]=size(B);
ny=size(C,1);
u0=f(1:nu);
y=f(nu+1:nu+ny);

xkk=xkk1+M*(y-C*xkk1);  % kalman

%% solver
p=[f(1:nu);xkk;f(ny+nu+1:2*ny+nu)];

b=S*p+s;
h=F*p;
%[zopt]=quadprog(H,h,G,b,[],[],[],[],[],options); % solve the optimal control problem
[zopt,time,iter] = wgsSolver(H,h,-G,-b,[],[],[],[],[],2);
feasRes=G*zopt-b;


nu=length(u0);
u=zopt(1:nu)+u0;

time = double(time);

xk1k=A*xkk1+B*u+L*(y-C*xkk1); % kalman

== matlab function mpc_tmpdemo2/MPC Controller/MPC/optimizer ==
  settings: updateMethod=DISCRETE  sampleTime=ts
  data: xk1 output BlockDataType; xk input BlockDataType; old_u input BlockDataType; ym input BlockDataType; ref input BlockDataType; md input BlockDataType; umin input BlockDataType; umax input BlockDataType; ymin input BlockDataType; ymax input BlockDataType; switch_in input BlockDataType; ext_mv input BlockDataType; MVtarget input BlockDataType; isQP parameter boolean; nx parameter BlockDataType; nu parameter BlockDataType; ny parameter BlockDataType; degrees parameter BlockDataType; Hinv parameter BlockDataType; Kx parameter BlockDataType; Ku1 parameter BlockDataType; Kut parameter BlockDataType; Kr parameter BlockDataType; Kv parameter BlockDataType; Mlim parameter BlockDataType; Mx parameter BlockDataType; Mu1 parameter BlockDataType; Mv parameter BlockDataType; z_degrees parameter BlockDataType; utarget parameter BlockDataType; p parameter BlockDataType; uoff parameter BlockDataType; voff parameter BlockDataType; yoff parameter BlockDataType; maxiter parameter BlockDataType; nxQP parameter BlockDataType; openloopflag parameter boolean; lims_inport parameter BlockDataType; no_umin parameter BlockDataType; no_umax parameter BlockDataType; no_ymin parameter BlockDataType; no_ymax parameter BlockDataType; switch_inport parameter BlockDataType; no_switch parameter BlockDataType; enable_value parameter BlockDataType; return_cost parameter BlockDataType; H parameter BlockDataType; return_sequence parameter BlockDataType; Linv parameter BlockDataType; Ac parameter BlockDataType; ywt input BlockDataType; uwt input BlockDataType; duwt input BlockDataType; rhoeps input BlockDataType; iA input boolean; u output BlockDataType; cost output BlockDataType; useq output BlockDataType; status output BlockDataType; xest output BlockDataType; no_ywt parameter BlockDataType; no_uwt parameter BlockDataType; no_duwt parameter BlockDataType; no_rhoeps parameter BlockDataType; Wy parameter BlockDataType; Wdu parameter BlockDataType; Jm parameter BlockDataType; SuJm parameter BlockDataType; Su1 parameter BlockDataType; Sx parameter BlockDataType; Hv parameter BlockDataType; Wu parameter BlockDataType; I1 parameter BlockDataType; iAout output boolean; A parameter BlockDataType; Bu parameter BlockDataType; Bv parameter BlockDataType; C parameter BlockDataType; Dv parameter BlockDataType; Mrows parameter BlockDataType; nCC parameter BlockDataType; Ecc parameter BlockDataType; Fcc parameter BlockDataType; Scc parameter BlockDataType; Gcc parameter BlockDataType; nv parameter BlockDataType; no_md parameter BlockDataType; no_ref parameter BlockDataType; no_uref parameter BlockDataType; no_mv parameter BlockDataType; Rscale parameter BlockDataType; MDscale parameter BlockDataType; myindex parameter BlockDataType; myoff parameter BlockDataType; xoff parameter BlockDataType; CustomEstimation parameter BlockDataType; M parameter BlockDataType; L parameter BlockDataType
function [xk1, u, cost, useq, status, xest, iAout] = fcn(...
            xk, old_u, ym, ref, md, umin, umax, ymin, ymax, switch_in, ext_mv, MVtarget, isQP, nx, nu, ny, degrees, Hinv, Kx, Ku1, Kut, Kr, Kv, Mlim, ...
            Mx, Mu1, Mv, z_degrees, utarget, p, uoff, voff, yoff, maxiter, nxQP, openloopflag, ...
            lims_inport, no_umin, no_umax, no_ymin, no_ymax, switch_inport, no_switch, enable_value, ...
            return_cost, H, return_sequence, Linv, Ac, ...
            ywt, uwt, duwt, rhoeps, iA, ...
            no_ywt, no_uwt, no_duwt, no_rhoeps,...
            Wy, Wdu, Jm, SuJm, Su1, Sx, Hv, Wu, I1, ...
            A, Bu, Bv, C, Dv, Mrows, nCC, Ecc, Fcc, Scc, Gcc, ...
            nv, no_md, no_ref, no_uref, no_mv, Rscale, MDscale, myindex, ...
            myoff, xoff, CustomEstimation, M, L)
%#codegen
coder.extrinsic('mpcblock_optimizer_double_mex');
coder.extrinsic('mpcblock_optimizer_single_mex');
coder.extrinsic('mpcblock_refmd_double_mex');
coder.extrinsic('mpcblock_refmd_single_mex');

% Parameters
isSimulation = coder.target('Sfun') && ~coder.target('RtwForRapid') && ~coder.target('RtwForSim');
isAdaptive = false;
isDouble = isa(ref,'double');
ZERO = zeros('like',ref);
ONE = ones('like',ref);

% Pre-allocate all the MEX block outputs for the simulation mode
%#ok<*NASGU>
%#ok<*PREALL>
if isSimulation
    rseq = zeros(p*ny,1,'like',ref); 
    vseq = zeros((p+1)*nv,1,'like',ref);
    v = zeros(nv,1,'like',ref);
    xk1 = zeros(nx,1,'like',ref);
    u = zeros(nu,1,'like',ref);
    cost =  ZERO;
    useq = zeros(p,nu,'like',ref); 
    status = ONE;
    xest = zeros(nx,1,'like',ref);
    iAout = iA;    
end

% Get reference and MD signals -- accounting for previewing
if isSimulation
    % When doing normal simulation in SL, use MEX for better compilation speed 
    if isDouble
        [rseq, vseq, v] = mpcblock_refmd_double_mex(ref,md,nv,ny,p,yoff,voff,no_md,no_ref,openloopflag, Rscale, MDscale);
    else
        [rseq, vseq, v] = mpcblock_refmd_single_mex(ref,md,nv,ny,p,yoff,voff,no_md,no_ref,openloopflag, Rscale, MDscale);        
    end
else
    % When doing code generation, use M code directly
    [rseq, vseq, v] = mpcblock_refmd(ref,md,nv,ny,p,yoff,voff,no_md,no_ref,openloopflag, Rscale, MDscale);
end

% External MV override.  
% NOTE: old_u and ext_mv input signals are dimensionless but include offset
old_u = old_u - uoff;
if no_mv==ONE
    delmv = zeros(nu,1,'like',ref);
else
    ext_mv = ext_mv - uoff;     % Bias correction
    delmv = ext_mv - old_u;
    old_u = ext_mv;
end

% Obtain x[k|k]
xk = xk - xoff; % Remove offset
if CustomEstimation==ONE
    % Input state is x(k|k)
    xest = xk(:);
else
    % Default state estimation.    
    % Scale measured output and remove offset.
    ym = ym.*Rscale(myindex) - myoff;
    % Correct x(k|k-1) for possible external mv override.
    % NOTE:  Offset was removed from x[k|k-1] at k=0.
    xk = xk + Bu*delmv;
    % Measurement upate to x(k|k)
    ym_est = C(myindex,:)*xk + Dv(myindex,:)*v;
    y_innov = ym - ym_est;
    xest = xk + M*y_innov;
end

% Real-time MV target override
% Note: utargetValue is a vector length p*nu.  
if no_uref==ONE
    % no external utarget
    utargetValue = utarget;
else
    % utarget is a vector length p*nu.  Define constant targets for the
    % entire horizon.
    MVtarget = MVtarget - uoff;         % Bias correction
    utargetValue = reshape(MVtarget(:,ones(p,1)),nu*p,1);
end

if isSimulation
    % When doing normal simulation in SL, use MEX for better compilation speed 
    if isDouble
        [u, cost, useq, status, iAout] = mpcblock_optimizer_double_mex(...
            rseq, vseq, umin, umax, ymin, ymax, switch_in, xest, old_u, iA, ...
            isQP, nu, ny, degrees, Hinv, Kx, Ku1, Kut, Kr, Kv, Mlim, ...
            Mx, Mu1, Mv, z_degrees, utargetValue, p, uoff, voff, yoff, maxiter, nxQP, openloopflag, ...
            lims_inport, no_umin, no_umax, no_ymin, no_ymax, switch_inport, ...
            no_switch, enable_value, return_cost, H, return_sequence, Linv, Ac, ...
            ywt, uwt, duwt, rhoeps, no_ywt, no_uwt, no_duwt, no_rhoeps,...
            Wy, Wdu, Jm, SuJm, Su1, Sx, Hv, Wu, I1, ...
            isAdaptive, A, Bu, Bv, C, Dv, ...
            Mrows, nCC, Ecc, Fcc, Scc, Gcc);    
    else
        [u, cost, useq, status, iAout] = mpcblock_optimizer_single_mex(...
            rseq, vseq, umin, umax, ymin, ymax, switch_in, xest, old_u, iA, ...
            isQP, nu, ny, degrees, Hinv, Kx, Ku1, Kut, Kr, Kv, Mlim, ...
            Mx, Mu1, Mv, z_degrees, utargetValue, p, uoff, voff, yoff, maxiter, nxQP, openloopflag, ...
            lims_inport, no_umin, no_umax, no_ymin, no_ymax, switch_inport, ...
            no_switch, enable_value, return_cost, H, return_sequence, Linv, Ac, ...
            ywt, uwt, duwt, rhoeps, no_ywt, no_uwt, no_duwt, no_rhoeps,...
            Wy, Wdu, Jm, SuJm, Su1, Sx, Hv, Wu, I1, ...
            isAdaptive, A, Bu, Bv, C, Dv, ...
            Mrows, nCC, Ecc, Fcc, Scc, Gcc);    
    end
else
    % When doing code generation, use M code directly
        [u, cost, useq, status, iAout] = mpcblock_optimizer(...
            rseq, vseq, umin, umax, ymin, ymax, switch_in, xest, old_u, iA, ...
            isQP, nu, ny, degrees, Hinv, Kx, Ku1, Kut, Kr, Kv, Mlim, ...
            Mx, Mu1, Mv, z_degrees, utargetValue, p, uoff, voff, yoff, maxiter, nxQP, openloopflag, ...
            lims_inport, no_umin, no_umax, no_ymin, no_ymax, switch_inport, ...
            no_switch, enable_value, return_cost, H, return_sequence, Linv, Ac, ...
            ywt, uwt, duwt, rhoeps, no_ywt, no_uwt, no_duwt, no_rhoeps,...
            Wy, Wdu, Jm, SuJm, Su1, Sx, Hv, Wu, I1, ...
            isAdaptive, A, Bu, Bv, C, Dv, ...
            Mrows, nCC, Ecc, Fcc, Scc, Gcc);    
end

if CustomEstimation==ONE
    xk1 = xk;
else
    % update x[k+1|k], assuming that above u and v will be applied.
    xk1 = A*xk + Bu*(u - uoff) + Bv*v + L*y_innov; 
end
xk1 = xk1 + xoff;   % Updated state must include offset

if CustomEstimation==ONE
    % sent to terminal
    xest = zeros(nx,1,'like',ref);
else
    xest = xest + xoff;
end

== matlab function mpc_tmpdemo2/QUADPROG/MATLAB Function ==
  data: f input; H input; F input; G input; S input; s input; u output; feasRes output; M input; L input; xk1k output; A input; B input; C input; xkk1 input; time output; iter output
%% solve the problem
%   min 0.5 z'Hz + h'z
%   s.t. Gz <= b

function [u,feasRes,xk1k,time,iter]=fcn(f,H,F,G,S,s,M,L,A,B,C,xkk1)
%% init
coder.extrinsic('tic');
coder.extrinsic('toc');
coder.extrinsic('quadprog');
coder.extrinsic('wgsSolver');
options.Algorithm='interior-point-convex';
options.MaxIter=1000;
options.TolCon=1.0000e-12; % default: 1e-8
options.TolFun=1.0000e-12; % default: 1e-8
options.TolX=1.0000e-12;   % default: 1e-8
options.Display='none';
zopt=zeros(size(H,1),1);
time = 0;
iter = 0;
mess = zeros(1,912);
mess = char(mess);
output.message = mess;
output.algorithm = 'interior-point-convex';
output.firstorderopt = 0;
output.constrviolation = 0;
output.iterations = 0;
output.cgiterations =[];

%% get info
[~,nu]=size(B);
ny=size(C,1);
u0=f(1:nu);
y=f(nu+1:nu+ny);

xkk=xkk1+M*(y-C*xkk1);  % kalman

%% solver
p=[f(1:nu);xkk;f(ny+nu+1:2*ny+nu)];

b=S*p+s;
h=F*p;
tic
[zopt,~,~,output]=quadprog(H,h,G,b,[],[],[],[],[],options); % solve the optimal control problem
%[zopt,~,~] = wgsSolver(H,h,-G,-b,[],[],[],[],[],1);
time = toc;
feasRes=G*zopt-b;
iter = output.iterations;

nu=length(u0);
u=zopt(1:nu)+u0;

xk1k=A*xkk1+B*u+L*(y-C*xkk1); % kalman
